simulink model "Injera_Dispensing_Manipulator"  (R2024a)
settings: Solver=ode4  StartTime=0.0  StopTime=16  FixedStep=1e-4  RelTol=1e-3
settings Model: Creator=ep710328  LastModifiedBy=ep710328

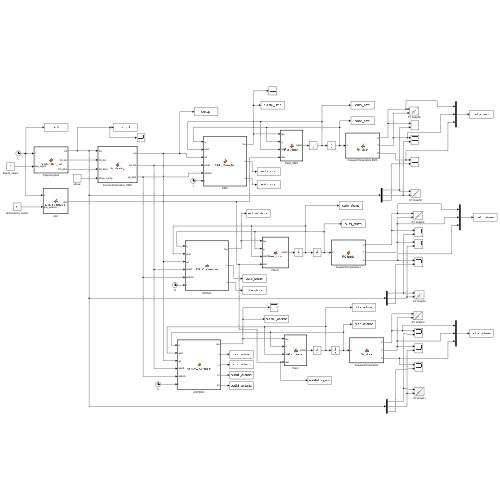
[thumbnail: Simulink's stored preview of the top-level diagram]
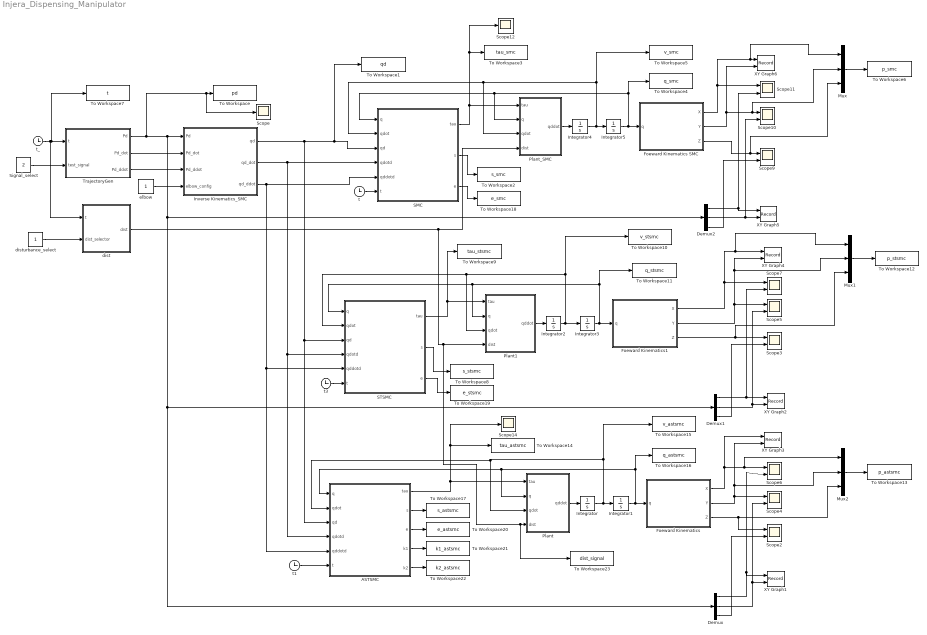
== system Injera_Dispensing_Manipulator ==
  ASTSMC : MATLAB Function  TreatAsAtomicUnit=on  SystemSampleTime=0.0001
  Demux : Demux  Outputs=3
  Demux1 : Demux  Outputs=3
  Demux2 : Demux  Outputs=3
  Foeward Kinematics : MATLAB Function  TreatAsAtomicUnit=on
  Foeward Kinematics SMC : MATLAB Function  TreatAsAtomicUnit=on
  Foeward Kinematics1 : MATLAB Function  TreatAsAtomicUnit=on
  Integrator : Integrator  InitialCondition=[0; 0; 0]
  Integrator1 : Integrator  InitialCondition=[1.5708; 2.0944; 0.05]
  Integrator2 : Integrator  InitialCondition=[0; 0; 0]
  Integrator3 : Integrator  InitialCondition=[1.5708; 2.0944; 0.05]
  Integrator4 : Integrator  InitialCondition=[0; 0; 0]
  Integrator5 : Integrator  InitialCondition=[1.5708; 2.0944; 0.05]
  Inverse Kinematics_SMC : MATLAB Function  TreatAsAtomicUnit=on
  Mux : Mux  Inputs=3
  Mux1 : Mux  Inputs=3
  Mux2 : Mux  Inputs=3
  Plant : MATLAB Function  TreatAsAtomicUnit=on
  Plant1 : MATLAB Function  TreatAsAtomicUnit=on
  Plant_SMC : MATLAB Function  TreatAsAtomicUnit=on
  SMC : MATLAB Function  TreatAsAtomicUnit=on  SystemSampleTime=0.0001
  STSMC : MATLAB Function  TreatAsAtomicUnit=on  SystemSampleTime=0.0001
  Scope : Scope
  Scope{2..7,9..11} (9 alike) : Scope  NumInputPorts=2
  Scope12 : Scope
  Scope14 : Scope
  Signal_select : Constant  Value=2
  To Workspace : ToWorkspace  VariableName=pd  SampleTime=-1
  To Workspace1 : ToWorkspace  VariableName=qd  SampleTime=-1
  To Workspace10 : ToWorkspace  VariableName=v_stsmc  SampleTime=-1
  To Workspace11 : ToWorkspace  VariableName=q_stsmc  SampleTime=-1
  To Workspace12 : ToWorkspace  VariableName=p_stsmc  SampleTime=-1
  To Workspace13 : ToWorkspace  VariableName=p_astsmc  SampleTime=-1
  To Workspace14 : ToWorkspace  VariableName=tau_astsmc  SampleTime=-1
  To Workspace15 : ToWorkspace  VariableName=v_astsmc  SampleTime=-1
  To Workspace16 : ToWorkspace  VariableName=q_astsmc  SampleTime=-1
  To Workspace17 : ToWorkspace  VariableName=s_astsmc  SampleTime=-1
  To Workspace18 : ToWorkspace  VariableName=e_smc  SampleTime=-1
  To Workspace19 : ToWorkspace  VariableName=e_stsmc  SampleTime=-1
  To Workspace2 : ToWorkspace  VariableName=s_smc  SampleTime=-1
  To Workspace20 : ToWorkspace  VariableName=e_astsmc  SampleTime=-1
  To Workspace21 : ToWorkspace  VariableName=k1_astsmc  SampleTime=-1
  To Workspace22 : ToWorkspace  VariableName=k2_astsmc  SampleTime=-1
  To Workspace23 : ToWorkspace  VariableName=dist_signal  SampleTime=-1
  To Workspace3 : ToWorkspace  VariableName=tau_smc  SampleTime=-1
  To Workspace4 : ToWorkspace  VariableName=q_smc  SampleTime=-1
  To Workspace5 : ToWorkspace  VariableName=v_smc  SampleTime=-1
  To Workspace6 : ToWorkspace  VariableName=p_smc  SampleTime=-1
  To Workspace7 : ToWorkspace  VariableName=t  SampleTime=-1
  To Workspace8 : ToWorkspace  VariableName=s_stsmc  SampleTime=-1
  To Workspace9 : ToWorkspace  VariableName=tau_stsmc  SampleTime=-1
  TrajectoryGen : MATLAB Function  TreatAsAtomicUnit=on
  XY Graph1 : Record  FileSettingsInternal="{\"entries\":[{\"content\":{\"excelSettings\":{\"content\":{},\"type\":\"Streamout.ExcelSettings\"}},\"type\":\"Streamout.FileSettingStorage\",\"uuid\":\"\"}],\"packageUris\":[\"http:\\/\\/schema.mathworks.com\\/mf0\\/streamout_blocks\\/R2020a\"],\"version\":\"1.0\"}"  Layout=[1 1]  SignalsInternal="{\"entries\":[{\"content\":{\"signals\":[{\"content\":{\"blockPath\":[],\"dimensions\":[1,1],\"domain\":\"\",\"lineColor\":\"#a2142f\",\"plots\":[ 1 ],\"port\":1,\"signalID\":1,\"signalName\":\"Demux:1\"},\"type\":\"RecordBlkView.Signal\",\"uuid\":\"\"},{\"content\":{\"blockPath\":[],\"dimensions\":[1,1],\"domain\":\"\",\"lineColor\":\"#139fff\",\"plots\":[ 1 ],\"port\":2,\"signalID\":2,\"signalName\":\"Demux:2\"},\"type\":\"RecordBlkView.Signal\",\"uuid\":\"\"}]},\"type\":\"RecordBlkView.InputSignals\",\"uuid\":\"\"}],\"packageUris\":[\"http:\\/\\/schema.mathworks.com\\/mf0\\/streamout_blocks\\/R2020a\"],\"version\":\"1.0\"}"  VisualizationBindings="{\"xyplotplugin\":{\"info\":[{\"series\":[{\"bindingParametersList\":[{\"parameter\":\"X-Axis\",\"signalID\":1,\"signalName\":\"Demux:1\"},{\"parameter\":\"Y-Axis\",\"signalID\":2,\"signalName\":\"Demux:2\"}],\"seriesID\":0}],\"subplotID\":1}]}}"  CompatibilityTag=XY
  XY Graph2 : Record  FileSettingsInternal="{\"entries\":[{\"content\":{\"excelSettings\":{\"content\":{},\"type\":\"Streamout.ExcelSettings\"}},\"type\":\"Streamout.FileSettingStorage\",\"uuid\":\"\"}],\"packageUris\":[\"http:\\/\\/schema.mathworks.com\\/mf0\\/streamout_blocks\\/R2020a\"],\"version\":\"1.0\"}"  Layout=[1 1]  SignalsInternal="{\"entries\":[{\"content\":{\"signals\":[{\"content\":{\"blockPath\":[],\"dimensions\":[1,1],\"domain\":\"\",\"lineColor\":\"#a2142f\",\"plots\":[ 1 ],\"port\":1,\"signalID\":1,\"signalName\":\"Demux1:1\"},\"type\":\"RecordBlkView.Signal\",\"uuid\":\"\"},{\"content\":{\"blockPath\":[],\"dimensions\":[1,1],\"domain\":\"\",\"lineColor\":\"#139fff\",\"plots\":[ 1 ],\"port\":2,\"signalID\":2,\"signalName\":\"Demux1:2\"},\"type\":\"RecordBlkView.Signal\",\"uuid\":\"\"}]},\"type\":\"RecordBlkView.InputSignals\",\"uuid\":\"\"}],\"packageUris\":[\"http:\\/\\/schema.mathworks.com\\/mf0\\/streamout_blocks\\/R2020a\"],\"version\":\"1.0\"}"  VisualizationBindings="{\"xyplotplugin\":{\"info\":[{\"series\":[{\"bindingParametersList\":[{\"parameter\":\"X-Axis\",\"signalID\":1,\"signalName\":\"Demux1:1\"},{\"parameter\":\"Y-Axis\",\"signalID\":2,\"signalName\":\"Demux1:2\"}],\"seriesID\":0}],\"subplotID\":1}]}}"  CompatibilityTag=XY
  XY Graph3 : Record  FileSettingsInternal="{\"entries\":[{\"content\":{\"excelSettings\":{\"content\":{},\"type\":\"Streamout.ExcelSettings\"}},\"type\":\"Streamout.FileSettingStorage\",\"uuid\":\"\"}],\"packageUris\":[\"http:\\/\\/schema.mathworks.com\\/mf0\\/streamout_blocks\\/R2020a\"],\"version\":\"1.0\"}"  Layout=[1 1]  SignalsInternal="{\"entries\":[{\"content\":{\"signals\":[{\"content\":{\"blockPath\":[],\"dimensions\":[1],\"domain\":\"\",\"lineColor\":\"#a2142f\",\"plots\":[ 1 ],\"port\":1,\"signalID\":1,\"signalName\":\"Foeward Kinematics:1\"},\"type\":\"RecordBlkView.Signal\",\"uuid\":\"\"},{\"content\":{\"blockPath\":[],\"dimensions\":[1],\"domain\":\"\",\"lineColor\":\"#139fff\",\"plots\":[ 1 ],\"port\":2,\"signalID\":2,\"signalName\":\"Foeward Kinematics:2\"},\"type\":\"RecordBlkView.Signal\",\"uuid\":\"\"}]},\"type\":\"RecordBlkView.InputSignals\",\"uuid\":\"\"}],\"packageUris\":[\"http:\\/\\/schema.mathworks.com\\/mf0\\/streamout_blocks\\/R2020a\"],\"version\":\"1.0\"}"  VisualizationBindings="{\"xyplotplugin\":{\"info\":[{\"series\":[{\"bindingParametersList\":[{\"parameter\":\"X-Axis\",\"signalID\":1,\"signalName\":\"Foeward Kinematics:1\"},{\"parameter\":\"Y-Axis\",\"signalID\":2,\"signalName\":\"Foeward Kinematics:2\"}],\"seriesID\":0}],\"subplotID\":1}]}}"  CompatibilityTag=XY
  XY Graph4 : Record  FileSettingsInternal="{\"entries\":[{\"content\":{\"excelSettings\":{\"content\":{},\"type\":\"Streamout.ExcelSettings\"}},\"type\":\"Streamout.FileSettingStorage\",\"uuid\":\"\"}],\"packageUris\":[\"http:\\/\\/schema.mathworks.com\\/mf0\\/streamout_blocks\\/R2020a\"],\"version\":\"1.0\"}"  Layout=[1 1]  SignalsInternal="{\"entries\":[{\"content\":{\"signals\":[{\"content\":{\"blockPath\":[],\"dimensions\":[1],\"domain\":\"\",\"lineColor\":\"#a2142f\",\"plots\":[ 1 ],\"port\":1,\"signalID\":1,\"signalName\":\"Foeward Kinematics1:1\"},\"type\":\"RecordBlkView.Signal\",\"uuid\":\"\"},{\"content\":{\"blockPath\":[],\"dimensions\":[1],\"domain\":\"\",\"lineColor\":\"#139fff\",\"plots\":[ 1 ],\"port\":2,\"signalID\":2,\"signalName\":\"Foeward Kinematics1:2\"},\"type\":\"RecordBlkView.Signal\",\"uuid\":\"\"}]},\"type\":\"RecordBlkView.InputSignals\",\"uuid\":\"\"}],\"packageUris\":[\"http:\\/\\/schema.mathworks.com\\/mf0\\/streamout_blocks\\/R2020a\"],\"version\":\"1.0\"}"  VisualizationBindings="{\"xyplotplugin\":{\"info\":[{\"series\":[{\"bindingParametersList\":[{\"parameter\":\"X-Axis\",\"signalID\":1,\"signalName\":\"Foeward Kinematics1:1\"},{\"parameter\":\"Y-Axis\",\"signalID\":2,\"signalName\":\"Foeward Kinematics1:2\"}],\"seriesID\":0}],\"subplotID\":1}]}}"  CompatibilityTag=XY
  XY Graph5 : Record  FileSettingsInternal="{\"entries\":[{\"content\":{\"excelSettings\":{\"content\":{},\"type\":\"Streamout.ExcelSettings\"}},\"type\":\"Streamout.FileSettingStorage\",\"uuid\":\"\"}],\"packageUris\":[\"http:\\/\\/schema.mathworks.com\\/mf0\\/streamout_blocks\\/R2020a\"],\"version\":\"1.0\"}"  Layout=[1 1]  SignalsInternal="{\"entries\":[{\"content\":{\"signals\":[{\"content\":{\"blockPath\":[],\"dimensions\":[1,1],\"domain\":\"\",\"lineColor\":\"#a2142f\",\"plots\":[ 1 ],\"port\":1,\"signalID\":1,\"signalName\":\"Demux2:1\"},\"type\":\"RecordBlkView.Signal\",\"uuid\":\"\"},{\"content\":{\"blockPath\":[],\"dimensions\":[1,1],\"domain\":\"\",\"lineColor\":\"#139fff\",\"plots\":[ 1 ],\"port\":2,\"signalID\":2,\"signalName\":\"Demux2:2\"},\"type\":\"RecordBlkView.Signal\",\"uuid\":\"\"}]},\"type\":\"RecordBlkView.InputSignals\",\"uuid\":\"\"}],\"packageUris\":[\"http:\\/\\/schema.mathworks.com\\/mf0\\/streamout_blocks\\/R2020a\"],\"version\":\"1.0\"}"  VisualizationBindings="{\"xyplotplugin\":{\"info\":[{\"series\":[{\"bindingParametersList\":[{\"parameter\":\"X-Axis\",\"signalID\":1,\"signalName\":\"Demux2:1\"},{\"parameter\":\"Y-Axis\",\"signalID\":2,\"signalName\":\"Demux2:2\"}],\"seriesID\":0}],\"subplotID\":1}]}}"  CompatibilityTag=XY
  XY Graph6 : Record  FileSettingsInternal="{\"entries\":[{\"content\":{\"excelSettings\":{\"content\":{},\"type\":\"Streamout.ExcelSettings\"}},\"type\":\"Streamout.FileSettingStorage\",\"uuid\":\"\"}],\"packageUris\":[\"http:\\/\\/schema.mathworks.com\\/mf0\\/streamout_blocks\\/R2020a\"],\"version\":\"1.0\"}"  Layout=[1 1]  SignalsInternal="{\"entries\":[{\"content\":{\"signals\":[{\"content\":{\"blockPath\":[],\"dimensions\":[1],\"domain\":\"\",\"lineColor\":\"#a2142f\",\"plots\":[ 1 ],\"port\":1,\"signalID\":1,\"signalName\":\"Foeward Kinematics SMC:1\"},\"type\":\"RecordBlkView.Signal\",\"uuid\":\"\"},{\"content\":{\"blockPath\":[],\"dimensions\":[1],\"domain\":\"\",\"lineColor\":\"#139fff\",\"plots\":[ 1 ],\"port\":2,\"signalID\":2,\"signalName\":\"Foeward Kinematics SMC:2\"},\"type\":\"RecordBlkView.Signal\",\"uuid\":\"\"}]},\"type\":\"RecordBlkView.InputSignals\",\"uuid\":\"\"}],\"packageUris\":[\"http:\\/\\/schema.mathworks.com\\/mf0\\/streamout_blocks\\/R2020a\"],\"version\":\"1.0\"}"  VisualizationBindings="{\"xyplotplugin\":{\"info\":[{\"series\":[{\"bindingParametersList\":[{\"parameter\":\"X-Axis\",\"signalID\":1,\"signalName\":\"Foeward Kinematics SMC:1\"},{\"parameter\":\"Y-Axis\",\"signalID\":2,\"signalName\":\"Foeward Kinematics SMC:2\"}],\"seriesID\":0}],\"subplotID\":1}]}}"  CompatibilityTag=XY
  dist : MATLAB Function  TreatAsAtomicUnit=on
  disturbance_select : Constant
  elbow : Constant
  t : Clock
  t1 : Clock
  t3 : Clock
  t_ : Clock
  wires:
  Integrator1/1 -> Foeward Kinematics/1(q), To Workspace16/1, Plant/2(q), ASTSMC/1(q)
  ASTSMC/1(tau) -> Plant/1(tau), Scope14/1, To Workspace14/1
  Integrator/1 -> Integrator1/1, To Workspace15/1, Plant/3(qdot), ASTSMC/2(qdot)
  Plant/1(qddot) -> Integrator/1
  dist/1(dist) -> To Workspace23/1, Plant/4(dist), Plant1/4(dist), Plant_SMC/4(dist)
  TrajectoryGen/1(Pd) -> Scope/1, To Workspace/1, Inverse Kinematics_SMC/1(Pd), Demux2/1, Demux1/1, Demux/1
  TrajectoryGen/2(Pd_dot) -> Inverse Kinematics_SMC/2(Pd_dot)
  TrajectoryGen/3(Pd_ddot) -> Inverse Kinematics_SMC/3(Pd_ddot)
  Inverse Kinematics_SMC/1(qd) -> To Workspace1/1, SMC/3(qd), STSMC/3(qd), ASTSMC/3(qd)
  Inverse Kinematics_SMC/2(qd_dot) -> SMC/4(qdotd), ASTSMC/4(qdotd), STSMC/4(qdotd)
  Inverse Kinematics_SMC/3(qd_ddot) -> SMC/5(qddotd), STSMC/5(qddotd), ASTSMC/5(qddotd)
  Demux/1 -> Scope6/2, XY Graph1/1
  Demux/2 -> Scope4/2, XY Graph1/2
  Demux/3 -> Scope2/2
  t1/1 -> ASTSMC/6(t)
  Demux1/3 -> Scope3/2
  Demux1/2 -> Scope5/2, XY Graph2/2
  STSMC/2(s) -> To Workspace8/1
  STSMC/1(tau) -> Plant1/1(tau), To Workspace9/1
  Demux1/1 -> Scope7/2, XY Graph2/1
  Integrator3/1 -> Plant1/2(q), STSMC/1(q), To Workspace11/1, Foeward Kinematics1/1(q)
  Plant1/1(qddot) -> Integrator2/1
  Integrator2/1 -> Plant1/3(qdot), STSMC/2(qdot), To Workspace10/1, Integrator3/1
  t3/1 -> STSMC/6(t)
  elbow/1 -> Inverse Kinematics_SMC/4(elbow_config)
  t/1 -> SMC/6(t)
  Foeward Kinematics SMC/3(Z) -> Mux/3, Scope9/1
  Signal_select/1 -> TrajectoryGen/2(test_signal)
  Integrator4/1 -> Integrator5/1, To Workspace5/1, Plant_SMC/3(qdot), SMC/2(qdot)
  Foeward Kinematics SMC/1(X) -> Scope11/1, Mux/1, XY Graph6/1
  Integrator5/1 -> Foeward Kinematics SMC/1(q), To Workspace4/1, Plant_SMC/2(q), SMC/1(q)
  SMC/2(s) -> To Workspace2/1
  t_/1 -> dist/1(t), TrajectoryGen/1(t), To Workspace7/1
  Demux2/1 -> XY Graph5/1, Scope11/2
  SMC/1(tau) -> Plant_SMC/1(tau), To Workspace3/1, Scope12/1
  Foeward Kinematics SMC/2(Y) -> Mux/2, Scope10/1, XY Graph6/2
  Demux2/2 -> XY Graph5/2, Scope10/2
  Demux2/3 -> Scope9/2
  Plant_SMC/1(qddot) -> Integrator4/1
  Mux/1 -> To Workspace6/1
  Mux1/1 -> To Workspace12/1
  Foeward Kinematics1/2(Y) -> Scope5/1, Mux1/2, XY Graph4/2
  Foeward Kinematics1/1(X) -> Scope7/1, Mux1/1, XY Graph4/1
  Foeward Kinematics1/3(Z) -> Scope3/1, Mux1/3
  Foeward Kinematics/3(Z) -> Mux2/3, Scope2/1
  Foeward Kinematics/1(X) -> Mux2/1, Scope6/1, XY Graph3/1
  Foeward Kinematics/2(Y) -> XY Graph3/2, Mux2/2, Scope4/1
  Mux2/1 -> To Workspace13/1
  SMC/3(e) -> To Workspace18/1
  STSMC/3(e) -> To Workspace19/1
  ASTSMC/2(s) -> To Workspace17/1
  ASTSMC/3(e) -> To Workspace20/1
  ASTSMC/4(k1) -> To Workspace21/1
  ASTSMC/5(k2) -> To Workspace22/1
  disturbance_select/1 -> dist/2(dist_selector)

== matlab function Injera_Dispensing_Manipulator/Foeward Kinematics SMC ==
  settings: updateMethod=DISCRETE
  data: q input; X output; Y output; Z output
function [X, Y, Z] = FK_block(q)
% Forward kinematics of the 3-DOF R-R-P SCARA manipulator
%
% Input:
%   q = [theta1; theta2; d3]
%
% Output:
%   X, Y, Z = End-effector Cartesian position

%% PARAMETERS
l1 = 0.40;    % Shoulder link length [m]
l2 = 0.35;    % Elbow link length [m]
d1 = 0.50;    % Fixed shoulder height [m]

%% JOINT VARIABLES
theta1 = q(1);
theta2 = q(2);
d3     = q(3);

%% FORWARD KINEMATICS
X = l1*cos(theta1) + l2*cos(theta1 + theta2);
Y = l1*sin(theta1) + l2*sin(theta1 + theta2);
Z = d3;

end

== matlab function Injera_Dispensing_Manipulator/Inverse Kinematics_SMC ==
  settings: updateMethod=DISCRETE
  data: Pd input; qd output; Pd_dot input; Pd_ddot input; elbow_config input; qd_dot output; qd_ddot output
function [qd, qd_dot, qd_ddot] = IK_Velocity(Pd, Pd_dot, Pd_ddot, elbow_config)
% Converts task-space position/velocity/acceleration vectors to joint-space
% via closed-form IK + analytic Jacobian. No numerical differentiation.
% Pd = [Xd;Yd;d3d], Pd_dot = [Xd_dot;Yd_dot;d3d_dot], Pd_ddot likewise.
% Outputs qd, qd_dot, qd_ddot = [theta1;theta2;d3] and derivatives.

%% ROBOT PARAMETERS -- must match IK_block/Plant_block
l1 = 0.40;
l2 = 0.35;

Xd = Pd(1); Yd = Pd(2); d3d = Pd(3);
Xd_dot = Pd_dot(1); Yd_dot = Pd_dot(2); d3d_dot = Pd_dot(3);
Xd_ddot = Pd_ddot(1); Yd_ddot = Pd_ddot(2); d3d_ddot = Pd_ddot(3);

%% INVERSE KINEMATICS -- position (matches IK_block, eq. 2.22-2.25)
r2 = Xd^2 + Yd^2;
if r2 > (l1+l2)^2 || r2 < (l1-l2)^2
    warning('IK_Velocity_block: target outside reachable annulus.');
end

c2 = (r2 - l1^2 - l2^2) / (2*l1*l2);
c2 = min(max(c2, -1), 1);

s2 = elbow_config * sqrt(1 - c2^2);
theta2 = atan2(s2, c2);
theta1 = atan2(Yd, Xd) - atan2(l2*sin(theta2), l1 + l2*cos(theta2));

qd = [theta1; theta2; d3d];

%% PLANAR JACOBIAN J(theta1,theta2): [Xdot;Ydot] = J*[theta1dot;theta2dot]
s1  = sin(theta1); c1 = cos(theta1);
s12 = sin(theta1+theta2); c12 = cos(theta1+theta2);

J = [-l1*s1 - l2*s12,  -l2*s12;
      l1*c1 + l2*c12,   l2*c12];

detJ = J(1,1)*J(2,2) - J(1,2)*J(2,1);
if abs(detJ) < 1e-6
    warning('IK_Velocity_block: near-singular Jacobian.');
end

%% JOINT VELOCITY
theta_dot = J \ [Xd_dot; Yd_dot];
theta1_dot = theta_dot(1);
theta2_dot = theta_dot(2);

qd_dot = [theta1_dot; theta2_dot; d3d_dot];

%% JACOBIAN TIME-DERIVATIVE
Jdot = [-l1*c1*theta1_dot - l2*c12*(theta1_dot+theta2_dot),  -l2*c12*(theta1_dot+theta2_dot);
        -l1*s1*theta1_dot - l2*s12*(theta1_dot+theta2_dot),  -l2*s12*(theta1_dot+theta2_dot)];

%% JOINT ACCELERATION
theta_ddot = J \ ([Xd_ddot; Yd_ddot] - Jdot*theta_dot);

qd_ddot = [theta_ddot(1); theta_ddot(2); d3d_ddot];

end

== matlab function Injera_Dispensing_Manipulator/Plant_SMC ==
  data: tau input; q input; qdot input; qddot output; dist input
function qddot = Plant_block(tau, q, qdot, dist)
% Forward dynamics: qddot = B^-1*(tau - C*qdot - G + dist)
% Matches manuscript eq. (3.6)-(3.8), (3.35)-(3.38); integrate externally
% MUST match SMC_Controller.m / STSMC_Controller.m / ASTSMC_Controller.m exactly

%% PARAMETERS
l1 = 0.40; l2 = 0.35;
lc1 = l1/2; lc2 = l2/2;
m1 = 4.5; m2 = 3.2; m3 = 4;
I1 = 0.05; I2 = 0.03; I3 = 0.001;
g = 9.81;

theta2 = q(2);
theta1dot = qdot(1);
theta2dot = qdot(2);

%% INERTIA MATRIX B(q)  -- eq (3.6)-(3.8), (3.38)
B11 = I1 + I2 + I3 + m1*lc1^2 + m2*(l1^2 + lc2^2 + 2*l1*lc2*cos(theta2)) ...
      + m3*(l1^2 + l2^2 + 2*l1*l2*cos(theta2));
B12 = I2 + I3 + m2*(lc2^2 + l1*lc2*cos(theta2)) + m3*(l2^2 + l1*l2*cos(theta2));
B22 = I2 + I3 + m2*lc2^2 + m3*l2^2;
B33 = m3;

B = [B11, B12, 0;
     B12, B22, 0;
     0,   0,   B33];

%% CORIOLIS/CENTRIFUGAL MATRIX C(q,qdot) -- eq (3.35)-(3.37), h per Christoffel derivation
h = (m2/2 + m3) * l1*l2*sin(theta2);
C = [-h*theta2dot, -h*(theta1dot + theta2dot), 0;
      h*theta1dot,  0,                          0;
      0,             0,                          0];

%% GRAVITY VECTOR G(q) -- eq (3.38)
G = [0; 0; m3*g];

%% FORWARD DYNAMICS
qddot = B \ (tau - C*qdot - G - dist);

end

== matlab function Injera_Dispensing_Manipulator/TrajectoryGen ==
  settings: updateMethod=DISCRETE
  data: t input; Pd output; Pd_dot output; Pd_ddot output; test_signal input
function [Pd, Pd_dot, Pd_ddot] = TrajectoryGen_Pos(t, test_signal)
% Task-space trajectory generator, multi-signal, vector I/O.
% test_signal (integer constant, wire a Constant block):
%   1 = Spiral   (Archimedean inward spiral, quintic time law)
%   2 = Step     (ideal step to a fixed target, qd_dot=qd_ddot=0 for t>0)
%   3 = Ramp     (point-to-point move, quintic S-curve blend, bounded jerk)
%   4 = Sinusoid (continuous oscillation, persistent excitation for tuning)
%
% Pd      = [Xd; Yd; d3d]            task-space position
% Pd_dot  = [Xd_dot; Yd_dot; d3d_dot]
% Pd_ddot = [Xd_ddot; Yd_ddot; d3d_ddot]
% d3d is JOINT-LEVEL prismatic command (no d1 offset) -- feeds straight
% into IK_Velocity_block; d1 belongs only in FK_block.

%% COMMON PARAMETERS (meters) -- adjust if your real values are in mm
R = 0.25; phi_max = 14*pi; b = R/phi_max;   % spiral, Eq. (2.27)
xc = 0.45; yc = 0;                          % pan center [m]
d3max = 0.20; d3min = 0.05;                 % prismatic stroke [m]
tf = 20;                                     % motion duration [s], shared by modes 1 & 3

% Start/target points for Step and Ramp (edit to your test case)
X0 = 0.45; Y0 = 0.25; d30 = 0.20;    % start point
Xf = 0.7; Yf = 0; d3f = 0.2;   % target point

% Sinusoid parameters (mode 4)
Ax = 0.10; Ay = 0.10; Ad3 = 0.05;    % amplitudes [m]
w  = 0.5;                            % angular frequency [rad/s]
d3_mid = (d3max+d3min)/2;

%% INITIALIZE (required so every branch produces consistent output sizes)
Xd=0; Yd=0; d3d=0; Xd_dot=0; Yd_dot=0; d3d_dot=0; Xd_ddot=0; Yd_ddot=0; d3d_ddot=0;

switch test_signal

    case 1  % ---------------- SPIRAL ----------------
        tt = min(max(t,0), tf);
        a3 =  10*phi_max/tf^3; a4 = -15*phi_max/tf^4; a5 = 6*phi_max/tf^5;
        phi      = a3*tt^3 + a4*tt^4 + a5*tt^5;
        phi_dot  = 3*a3*tt^2 + 4*a4*tt^3 + 5*a5*tt^4;
        phi_ddot = 6*a3*tt + 12*a4*tt^2 + 20*a5*tt^3;

        r      = R - b*phi;
        r_dot  = -b*phi_dot;
        r_ddot = -b*phi_ddot;

        k = (d3max-d3min)/phi_max;
        d3d      = d3max - k*phi;
        d3d_dot  = -k*phi_dot;
        d3d_ddot = -k*phi_ddot;

        Xd = xc + r*cos(phi);
        Yd = yc + r*sin(phi);
        Xd_dot = r_dot*cos(phi) - r*sin(phi)*phi_dot;
        Yd_dot = r_dot*sin(phi) + r*cos(phi)*phi_dot;
        Xd_ddot = r_ddot*cos(phi) - 2*r_dot*sin(phi)*phi_dot ...
                  - r*cos(phi)*phi_dot^2 - r*sin(phi)*phi_ddot;
        Yd_ddot = r_ddot*sin(phi) + 2*r_dot*cos(phi)*phi_dot ...
                  - r*sin(phi)*phi_dot^2 + r*cos(phi)*phi_ddot;

    case 2  % ---------------- STEP ----------------
        Xd = Xf; Yd = Yf; d3d = d3f;
        Xd_dot = 0; Yd_dot = 0; d3d_dot = 0;
        Xd_ddot = 0; Yd_ddot = 0; d3d_ddot = 0;

    case 3  % ---------------- RAMP (point-to-point, quintic S-curve) ----------------
        tt = min(max(t,0), tf);
        a3 = 10/tf^3; a4 = -15/tf^4; a5 = 6/tf^5;   % s(t): 0->1, s_dot=s_ddot=0 at both ends
        s      = a3*tt^3 + a4*tt^4 + a5*tt^5;
        s_dot  = 3*a3*tt^2 + 4*a4*tt^3 + 5*a5*tt^4;
        s_ddot = 6*a3*tt + 12*a4*tt^2 + 20*a5*tt^3;

        Xd = X0 + (Xf-X0)*s;      Xd_dot = (Xf-X0)*s_dot;      Xd_ddot = (Xf-X0)*s_ddot;
        Yd = Y0 + (Yf-Y0)*s;      Yd_dot = (Yf-Y0)*s_dot;      Yd_ddot = (Yf-Y0)*s_ddot;
        d3d = d30 + (d3f-d30)*s;  d3d_dot = (d3f-d30)*s_dot;   d3d_ddot = (d3f-d30)*s_ddot;

    case 4  % ---------------- SINUSOID (persistent excitation) ----------------
        Xd = xc + Ax*sin(w*t);
        Yd = yc + Ay*cos(w*t);
        d3d = d3_mid + Ad3*sin(w*t);

        Xd_dot = Ax*w*cos(w*t);
        Yd_dot = -Ay*w*sin(w*t);
        d3d_dot = Ad3*w*cos(w*t);

        Xd_ddot = -Ax*w^2*sin(w*t);
        Yd_ddot = -Ay*w^2*cos(w*t);
        d3d_ddot = -Ad3*w^2*sin(w*t);

    otherwise
        warning('TrajectoryGen_Pos: unknown test_signal=%d, defaulting to spiral.', test_signal);
        % falls through with all zeros initialized above -- edit if you'd
        % rather this silently default to case 1 logic instead
end

%% ASSEMBLE OUTPUT VECTORS
Pd      = [Xd;      Yd;      d3d];
Pd_dot  = [Xd_dot;  Yd_dot;  d3d_dot];
Pd_ddot = [Xd_ddot; Yd_ddot; d3d_ddot];

end

== matlab function Injera_Dispensing_Manipulator/STSMC ==
  settings: updateMethod=DISCRETE
  data: q input; tau output; qdot input; qd input; qdotd input; qddotd input; t input; s output; e output
function [tau, s, e] = STSMC_Controller(q, qdot, qd, qdotd, qddotd, t)
% Super-Twisting Sliding Mode Controller -- FIXED GAINS (no adaptation)
% Same structure as ASTSMC_Controller but k1, k2 are constants.
% Used for comparison against ASTSMC (isolates the value of adaptation).

%% PARAMETERS
Lambda = diag([5 5 5]);      % sliding surface gain, eq (4.6)
k1_fix = [5; 5; 5];           % FIXED first-stage gain (tune by hand)
beta_c = 2;                    % coupling constant, K2=(beta_c/2)K1^2
k2_fix = (beta_c/2) * k1_fix.^2;  % FIXED second-stage gain, algebraic
phi    = [0.01; 0.01; 0.01];  % boundary-layer width, eq (4.18)
Te     = 0.001;                % nominal sample period for dt fallback

% Plant params -- MUST match Plant_block.m and SMC_Controller.m exactly
l1 = 0.40; l2 = 0.35; lc1 = l1/2; lc2 = l2/2;
m1 = 4.5; m2 = 3.2; m3 = 4;
I1 = 0.05; I2 = 0.03; I3 = 0.001;
g = 9.81;

%% PERSISTENT STATES -- only v (super-twisting integral), no k1/w/adaptation
persistent v last_t initialized
if isempty(initialized)
    v = zeros(3,1);
    last_t = t;
    initialized = true;
end

dt = t - last_t;
if dt <= 0 || dt > 1
    dt = Te;
end

%% ERROR AND SLIDING SURFACE -- eq (4.4)-(4.6)
e    = qd - q;
edot = qdotd - qdot;
s    = edot + Lambda*e;

%% MODEL MATRICES B(q), C(q,qdot), G(q) -- must match Plant_block.m
theta2 = q(2); theta1dot = qdot(1); theta2dot = qdot(2);

B11 = I1 + I2 + I3 + m1*lc1^2 + m2*(l1^2 + lc2^2 + 2*l1*lc2*cos(theta2)) ...
      + m3*(l1^2 + l2^2 + 2*l1*l2*cos(theta2));
B12 = I2 + I3 + m2*(lc2^2 + l1*lc2*cos(theta2)) + m3*(l2^2 + l1*l2*cos(theta2));
B22 = I2 + I3 + m2*lc2^2 + m3*l2^2;
B33 = m3;
B = [B11, B12, 0; B12, B22, 0; 0, 0, B33];

h = (m2/2 + m3) * l1*l2*sin(theta2);
C = [-h*theta2dot, -h*(theta1dot+theta2dot), 0;
      h*theta1dot,  0,                        0;
      0,             0,                        0];
G = [0; 0; m3*g];

%% EQUIVALENT CONTROL -- eq (4.15), unchanged
tau_eq = B*(qddotd + Lambda*edot) + C*qdot + G;

%% SWITCHING CONTROL -- eq (4.18), fixed k1/k2 instead of adaptive
tau_sw = B*(k1_fix .* sqrt(abs(s)) .* tanh(s./phi) - v);

%% TOTAL CONTROL LAW
tau = tau_eq + tau_sw;

%% AUXILIARY STATE UPDATE -- eq (4.19), fixed k2
vdot = -k2_fix .* tanh(s./phi);
v = v + vdot*dt;

%% UPDATE TIME
last_t = t;

end

== matlab function Injera_Dispensing_Manipulator/Foeward Kinematics1 ==
  settings: updateMethod=DISCRETE
  data: q input; X output; Y output; Z output
function [X, Y, Z] = FK_block(q)
% Forward kinematics of the 3-DOF R-R-P SCARA manipulator
%
% Input:
%   q = [theta1; theta2; d3]
%
% Output:
%   X, Y, Z = End-effector Cartesian position

%% PARAMETERS
l1 = 0.40;    % Shoulder link length [m]
l2 = 0.35;    % Elbow link length [m]
d1 = 0.50;    % Fixed shoulder height [m]

%% JOINT VARIABLES
theta1 = q(1);
theta2 = q(2);
d3     = q(3);

%% FORWARD KINEMATICS
X = l1*cos(theta1) + l2*cos(theta1 + theta2);
Y = l1*sin(theta1) + l2*sin(theta1 + theta2);
Z = d3;

end

== matlab function Injera_Dispensing_Manipulator/dist ==
  data: t input; dist output; dist_selector input
function dist = DisturbanceGen(t, dist_selector)
% Lumped matched disturbance Delta(q,qdot,t), eq (4.2): must be
% continuously differentiable with bounded derivative (Assumption 1).
% dist_selector (integer constant):
%   1 = None       (zero -- nominal/baseline run)
%   2 = Step       (smoothed onset -- true step violates Assumption 1's
%                    differentiability requirement, so this uses a fast
%                    tanh-based ramp instead of an ideal discontinuity)
%   3 = Sinusoidal (smooth, gated to activate at t_on -- represents
%                    cyclic batter-viscosity variation once dispensing
%                    is underway, not from t=0)
%   4 = Combined   (step-onset + sinusoidal -- worst-case test)
%   5 = Pulse      (smoothed rectangular pulse -- transient rejection test)
%
% ALL non-zero modes are gated to activate at the SAME onset time t_on,
% so switching dist_selector for different tests never changes when the
% disturbance actually starts -- disturbance is exactly ~0 for t<t_on
% and smoothly ramps in at t=t_on for every mode.

%% PARAMETERS
t_on   = 5;         % disturbance onset time [s] -- applies to ALL modes
t_off  = 15;         % pulse end time [s], mode 5 only
r      = 50;          % smoothing sharpness for tanh-based edges (higher = sharper)

% Magnitudes -- match torque/force units: [N.m; N.m; N] for [tau1;tau2;F3]
step_mag  = [2; 2; 2.0];
sin_mag   = [0.3; 0.2; 1.0];
sin_freq  = 2*pi*0.3;                 % 0.3 Hz
pulse_mag = [0.6; 0.5; 2.5];

%% COMMON ONSET GATE (shared by every mode for consistent t=5s activation)
onset = 0.5*(1 + tanh(r*(t - t_on)));

%% GENERATE PER MODE
switch dist_selector
    case 1  % None
        dist = zeros(3,1);

    case 2  % Step (smoothed onset, satisfies bounded-derivative assumption)
        dist = step_mag .* onset;

    case 3  % Sinusoidal, gated at t_on (was previously active from t=0 -- fixed)
        dist = sin_mag .* sin(sin_freq * t) .* onset;

    case 4  % Combined: smoothed step onset + sinusoidal, superimposed
        dist = step_mag.*onset + sin_mag.*sin(sin_freq*t).*onset;

    case 5  % Smoothed rectangular pulse (transient rejection test)
        offset = 0.5*(1 + tanh(r*(t_off - t)));
        dist = pulse_mag .* onset .* offset;

    otherwise
        warning('DisturbanceGen: unknown dist_selector=%d, using zero.', dist_selector);
        dist = zeros(3,1);
end

end

== matlab function Injera_Dispensing_Manipulator/ASTSMC ==
  settings: updateMethod=DISCRETE
  data: q input; tau output; qdot input; qd input; qdotd input; qddotd input; t input; s output; e output; k1 output; k2 output
function [tau,s,e,k1,k2] = ASTSMC_Controller(q,qdot,qd,qdotd,qddotd,t)
%#codegen
% Adaptive Super-Twisting Sliding Mode Controller
% Simulink MATLAB Function Block Compatible (R2021-R2025)
%% ===================== PARAMETERS ==========================
Lambda = diag([5 5 5]);
beta_c = 2;
beta1  = [2; 2; 4];
alpha_s = [8; 8; 3];
k_min = [3; 3; 1.5];
k_max = [50; 50; 20];
tau_f = 0.01;
Te    = 0.001;
phi = [0.01; 0.01; 0.03];
%% Robot Parameters -- MUST match Plant_block.m and SMC/STSMC_Controller.m exactly
l1 = 0.40;
l2 = 0.35;
lc1 = l1/2;
lc2 = l2/2;
m1 = 4.5;
m2 = 3.2;
m3 = 4;
I1 = 0.05;
I2 = 0.03;
I3 = 0.001;
g = 9.81;
%% ================= OUTPUT PREALLOCATION ====================
tau = zeros(3,1);
s   = zeros(3,1);
e   = zeros(3,1);
k1  = zeros(3,1);
k2  = zeros(3,1);
%% ================= PERSISTENT STATES =======================
persistent k1_state
persistent v_state
persistent w_state
persistent last_t
if isempty(k1_state)
    k1_state = 5 * ones(3,1);
    v_state = zeros(3,1);
    w_state = zeros(3,1);
    last_t = t;
end
%% Time step
dt = t-last_t;
if (dt<=0)||(dt>1)
    dt = Te;
end
%% ================= Tracking Error ==========================
e = qd-q;
edot = qdotd-qdot;
s = edot + Lambda*e;
%% ================= Differentiator ==========================
s_hat = (s-w_state)/tau_f;
psi = -s_hat;
wdot = (s-w_state)/tau_f;
w_state = w_state + dt*wdot;
%% ================= Adaptive Gain ===========================
% NOTE: alpha_s is now a 3x1 per-axis vector -- must use .* (elementwise),
% not * (matrix multiplication), against the 3x1 (k1_state.*sqrt(abs(s))+abs(psi)) term.
alpha_t = alpha_s.*(k1_state.*sqrt(abs(s))+abs(psi));
K2_temp = (beta_c/2)*(k1_state.^2);
eps_t = (alpha_t + abs(psi) + abs(v_state))*Te + K2_temp*Te^2;
eps_t = max(eps_t,1e-6);
%% ================= Gain Update =============================
% NOTE: beta1 and k_min are now 3x1 per-axis vectors -- must index by i
% here, same as alpha_t/eps_t/psi/s, not used as scalars.
k1dot = zeros(3,1);
for i=1:3
    if abs(s(i))>eps_t(i)
        k1dot(i) = alpha_t(i)/(abs(psi(i))+eps_t(i));
    else
        k1dot(i) = -beta1(i)*(k1_state(i)-k_min(i));
    end
end
k1_state = k1_state + dt*k1dot;
k1_state = min(max(k1_state,k_min),k_max);
k2 = (beta_c/2)*(k1_state.^2);
%% ================= Robot Dynamics ==========================
theta2 = q(2);
theta1dot = qdot(1);
theta2dot = qdot(2);
B11 = I1+I2+I3 ...
    +m1*lc1^2 ...
    +m2*(l1^2+lc2^2+2*l1*lc2*cos(theta2)) ...
    +m3*(l1^2+l2^2+2*l1*l2*cos(theta2));
B12 = I2+I3 ...
    +m2*(lc2^2+l1*lc2*cos(theta2)) ...
    +m3*(l2^2+l1*l2*cos(theta2));
B22 = I2+I3+m2*lc2^2+m3*l2^2;
B33 = m3;
B = [B11 B12 0;
     B12 B22 0;
     0   0   B33];
h = (m2/2+m3)*l1*l2*sin(theta2);
C = [-h*theta2dot      -h*(theta1dot+theta2dot)    0;
      h*theta1dot       0                          0;
      0                 0                          0];
G = [0;
     0;
     m3*g];
%% ================= Equivalent Control ======================
tau_eq = B*(qddotd + Lambda*edot) + C*qdot + G;
%% ================= Switching Control =======================
tau_sw = B*(k1_state.*sqrt(abs(s)).*tanh(s./phi) - v_state);
%% ================= Total Control ===========================
tau = tau_eq + tau_sw;
%% ================= Super-Twisting Update ===================
vdot = -k2.*tanh(s./phi);
v_state = v_state + dt*vdot;
%% ================= Outputs ================================
k1 = k1_state;
last_t = t;
end

== matlab function Injera_Dispensing_Manipulator/Foeward Kinematics ==
  settings: updateMethod=DISCRETE
  data: q input; X output; Y output; Z output
function [X, Y, Z] = FK_block(q)
% Forward kinematics of the 3-DOF R-R-P SCARA manipulator
%
% Input:
%   q = [theta1; theta2; d3]
%
% Output:
%   X, Y, Z = End-effector Cartesian position

%% PARAMETERS
l1 = 0.40;    % Shoulder link length [m]
l2 = 0.35;    % Elbow link length [m]
d1 = 0.50;    % Fixed shoulder height [m]

%% JOINT VARIABLES
theta1 = q(1);
theta2 = q(2);
d3     = q(3);

%% FORWARD KINEMATICS
X = l1*cos(theta1) + l2*cos(theta1 + theta2);
Y = l1*sin(theta1) + l2*sin(theta1 + theta2);
Z = d3;

end

== matlab function Injera_Dispensing_Manipulator/Plant1 ==
  data: tau input; q input; qdot input; qddot output; dist input
function qddot = Plant_block(tau, q, qdot, dist)
% Forward dynamics: qddot = B^-1*(tau - C*qdot - G + dist)
% Matches manuscript eq. (3.6)-(3.8), (3.35)-(3.38); integrate externally
% MUST match SMC_Controller.m / STSMC_Controller.m / ASTSMC_Controller.m exactly

%% PARAMETERS
l1 = 0.40; l2 = 0.35;
lc1 = l1/2; lc2 = l2/2;
m1 = 4.5; m2 = 3.2; m3 = 4;
I1 = 0.05; I2 = 0.03; I3 = 0.001;
g = 9.81;

theta2 = q(2);
theta1dot = qdot(1);
theta2dot = qdot(2);

%% INERTIA MATRIX B(q)  -- eq (3.6)-(3.8), (3.38)
B11 = I1 + I2 + I3 + m1*lc1^2 + m2*(l1^2 + lc2^2 + 2*l1*lc2*cos(theta2)) ...
      + m3*(l1^2 + l2^2 + 2*l1*l2*cos(theta2));
B12 = I2 + I3 + m2*(lc2^2 + l1*lc2*cos(theta2)) + m3*(l2^2 + l1*l2*cos(theta2));
B22 = I2 + I3 + m2*lc2^2 + m3*l2^2;
B33 = m3;

B = [B11, B12, 0;
     B12, B22, 0;
     0,   0,   B33];

%% CORIOLIS/CENTRIFUGAL MATRIX C(q,qdot) -- eq (3.35)-(3.37), h per Christoffel derivation
h = (m2/2 + m3) * l1*l2*sin(theta2);
C = [-h*theta2dot, -h*(theta1dot + theta2dot), 0;
      h*theta1dot,  0,                          0;
      0,             0,                          0];

%% GRAVITY VECTOR G(q) -- eq (3.38)
G = [0; 0; m3*g];

%% FORWARD DYNAMICS
qddot = B \ (tau - C*qdot - G - dist);

end

== matlab function Injera_Dispensing_Manipulator/Plant ==
  data: tau input; q input; qdot input; qddot output; dist input
function qddot = Plant_block(tau, q, qdot, dist)
% Forward dynamics: qddot = B^-1*(tau - C*qdot - G + dist)
% Matches manuscript eq. (3.6)-(3.8), (3.35)-(3.38); integrate externally
% MUST match SMC_Controller.m / STSMC_Controller.m / ASTSMC_Controller.m exactly

%% PARAMETERS
l1 = 0.40; l2 = 0.35;
lc1 = l1/2; lc2 = l2/2;
m1 = 4.5; m2 = 3.2; m3 = 4;
I1 = 0.05; I2 = 0.03; I3 = 0.001;
g = 9.81;

theta2 = q(2);
theta1dot = qdot(1);
theta2dot = qdot(2);

%% INERTIA MATRIX B(q)  -- eq (3.6)-(3.8), (3.38)
B11 = I1 + I2 + I3 + m1*lc1^2 + m2*(l1^2 + lc2^2 + 2*l1*lc2*cos(theta2)) ...
      + m3*(l1^2 + l2^2 + 2*l1*l2*cos(theta2));
B12 = I2 + I3 + m2*(lc2^2 + l1*lc2*cos(theta2)) + m3*(l2^2 + l1*l2*cos(theta2));
B22 = I2 + I3 + m2*lc2^2 + m3*l2^2;
B33 = m3;

B = [B11, B12, 0;
     B12, B22, 0;
     0,   0,   B33];

%% CORIOLIS/CENTRIFUGAL MATRIX C(q,qdot) -- eq (3.35)-(3.37), h per Christoffel derivation
h = (m2/2 + m3) * l1*l2*sin(theta2);
C = [-h*theta2dot, -h*(theta1dot + theta2dot), 0;
      h*theta1dot,  0,                          0;
      0,             0,                          0];

%% GRAVITY VECTOR G(q) -- eq (3.38)
G = [0; 0; m3*g];

%% FORWARD DYNAMICS
qddot = B \ (tau - C*qdot - G - dist);

end

== matlab function Injera_Dispensing_Manipulator/SMC ==
  settings: updateMethod=DISCRETE
  data: q input; tau output; qdot input; qd input; qdotd input; qddotd input; t input; s output; e output
function [tau, s, e] = SMC_Controller(q, qdot, qd, qdotd, qddotd, t)
% Classical (first-order) Sliding Mode Controller -- discontinuous sign()
% This is the TRUE classical SMC baseline (chattering by design) --
% no boundary layer smoothing, no super-twisting, no adaptation.

%% PARAMETERS
Lambda = diag([5 5 5]);      % sliding surface gain, eq (4.6)
K_fix  = [10; 10; 10];        % FIXED switching gain (tune by hand)

% Plant params -- MUST match Plant_block.m exactly
l1 = 0.40; l2 = 0.35; lc1 = l1/2; lc2 = l2/2;
m1 = 4.5; m2 = 3.2; m3 = 4;
I1 = 0.05; I2 = 0.03; I3 = 0.001;
g = 9.81;

%% ERROR AND SLIDING SURFACE -- eq (4.4)-(4.6)
e    = qd - q;
edot = qdotd - qdot;
s    = edot + Lambda*e;

%% MODEL MATRICES B(q), C(q,qdot), G(q) -- must match Plant_block.m
theta2 = q(2); theta1dot = qdot(1); theta2dot = qdot(2);

B11 = I1 + I2 + I3 + m1*lc1^2 + m2*(l1^2 + lc2^2 + 2*l1*lc2*cos(theta2)) ...
      + m3*(l1^2 + l2^2 + 2*l1*l2*cos(theta2));
B12 = I2 + I3 + m2*(lc2^2 + l1*lc2*cos(theta2)) + m3*(l2^2 + l1*l2*cos(theta2));
B22 = I2 + I3 + m2*lc2^2 + m3*l2^2;
B33 = m3;
B = [B11, B12, 0; B12, B22, 0; 0, 0, B33];

h = (m2/2 + m3) * l1*l2*sin(theta2);
C = [-h*theta2dot, -h*(theta1dot+theta2dot), 0;
      h*theta1dot,  0,                        0;
      0,             0,                        0];
G = [0; 0; m3*g];

%% EQUIVALENT CONTROL -- eq (4.15), unchanged
tau_eq = B*(qddotd + Lambda*edot) + C*qdot + G;

%% SWITCHING CONTROL -- discontinuous sign() (true classical SMC)
tau_sw = B*(K_fix .* sign(s));

%% TOTAL CONTROL LAW
tau = tau_eq + tau_sw;

end
